simulink model "MSAP_avec_obs"  (R2021a)
settings: Solver=VariableStepAuto  StartTime=0.0  StopTime=10  FixedStep=0.00000001  RelTol=1e-4
values from neighbouring files (symbols this model uses):
  B = [ 1/Ld 0 ... (first row only)    [script_projet.m]
  C = [1 0 0 0 ... (first row only)    [script_projet.m]
  Cr = 5    [script_projet.m]
  f = 14*10^-5    (= 0.00014)    [script_projet.m]
  J = 11*10^-5    (= 0.00011)    [script_projet.m]
  Kid = 3*Rs/trd    (= 0.0014)    [script_projet.m]
  KiO = 3*f/tr2    (= 0.00011)    [script_projet.m]
  Kiq = 3*Rs/trq    (= 0.0028)    [script_projet.m]
  Kpd = 3*Ld/trd    (= 3.26666666667e-06)    [script_projet.m]
  KpO = 3*J/tr2*10^8    (= 8642.85714286)    [script_projet.m]
  Kpq = 3*Lq/trq    (= 1.30666666667e-05)    [script_projet.m]
  Ld = 0.0014    [script_projet.m]
  Lq = 0.0028    [script_projet.m]
  P = 4    [script_projet.m]
  phi_f = 0.12    [script_projet.m]
  Q = [1 0 0 0 ... (first row only)    [script_projet.m]
  R = [1 0 ... (first row only)    [script_projet.m]
  Rs = 0.6    [script_projet.m]
libraries: simulink x1
settings Model: Creator=atestard2020  LastModifiedBy=atestard2020
settings SolverCC: MaxConsecutiveMinStep=1000

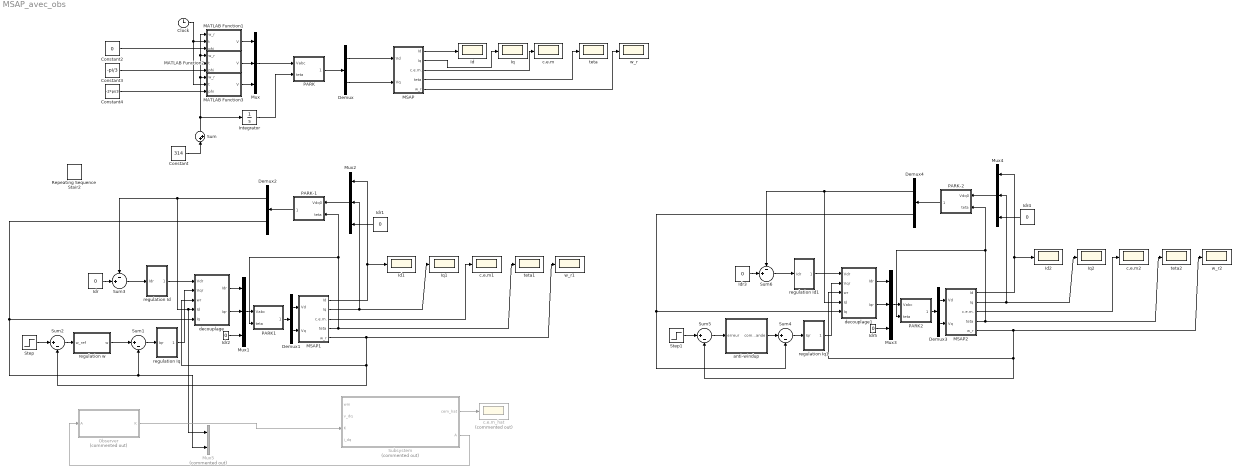
== system MSAP_avec_obs ==
  Clock : Clock
      settings: Decimation=1000000
  Constant : Constant  Value=314
  Constant2 : Constant  Value=0
  Constant3 : Constant  Value=-pi/3
  Constant4 : Constant  Value=-2*pi/3
  Demux{,1..4} (5 alike) : Demux  Outputs=2
  Id : Scope
  Id1 : Scope
  Id2 : Scope
  Idr{,1..5} (6 alike) : Constant  Value=0
  Integrator : Integrator
  Iq : Scope
  Iq1 : Scope
  Iq2 : Scope
  MATLAB Function1 : MATLAB Function  TreatAsAtomicUnit=on
  MATLAB Function2 : MATLAB Function  TreatAsAtomicUnit=on
  MATLAB Function3 : MATLAB Function  TreatAsAtomicUnit=on
  MSAP : Subsystem
  MSAP1 : Subsystem
  MSAP2 : Subsystem
  Mux{,1..4} (5 alike) : Mux  Inputs=3
  Mux5 : Mux  Commented=on  Inputs=2
  Observer : Subsystem  Commented=on
  PARK : MATLAB Function  TreatAsAtomicUnit=on
  PARK-1 : MATLAB Function  TreatAsAtomicUnit=on
  PARK-2 : MATLAB Function  TreatAsAtomicUnit=on
  PARK1 : MATLAB Function  TreatAsAtomicUnit=on
  PARK2 : MATLAB Function  TreatAsAtomicUnit=on
  Repeating Sequence Stair2 : simulink/Sources/Repeating Sequence Stair  OutValues=[3 1 4 2 1].'  tsamp=0.4  OutMin=[]  OutMax=[]  OutDataTypeStr=double  OutputDataTypeScalingMode=double  OutDataType=fixdt(0,8)  ConRadixGroup=Best Precision: Vector-wise  OutScaling=2^-12
  Step : Step  After=4  SampleTime=0
  Step1 : Step  SampleTime=0
  Subsystem : Subsystem  Commented=on
  Sum : Sum  Inputs=|++
  Sum{1..2,4..5} (4 alike) : Sum  Inputs=|+-
  Sum3 : Sum  Inputs=-+|
  Sum6 : Sum  Inputs=-+|
  anti-windup : Subsystem
  c.e.m : Scope
  c.e.m1 : Scope
  c.e.m2 : Scope
  c.e.m_hat : Scope  Commented=on
  decouplage : Subsystem
  decouplage1 : Subsystem
  regulation Id : Subsystem
  regulation Id1 : Subsystem
  regulation Iq : Subsystem
  regulation Iq1 : Subsystem
  regulation w : Subsystem
  teta : Scope
  teta1 : Scope
  teta2 : Scope
  w_r : Scope
  w_r1 : Scope
  w_r2 : Scope
  wires:
  MATLAB Function1/1(V) -> Mux/1
  MATLAB Function2/1(V) -> Mux/2
  Integrator/1 -> PARK/2(teta)
  Mux/1 -> PARK/1(Vabc)
  Demux/1 -> MSAP/1(Vd)
  MATLAB Function3/1(V) -> Mux/3
  PARK/1(TVdq0) -> Demux/1
  Demux/2 -> MSAP/2(Vq)
  MSAP/4(teta) -> teta/1
  MSAP/5(w_r) -> w_r/1
  MSAP/3(c.e.m.) -> c.e.m/1
  MSAP/2(Iq) -> Iq/1
  MSAP/1(Id) -> Id/1
  Constant2/1 -> MATLAB Function1/3(phi)
  Constant3/1 -> MATLAB Function2/3(phi)
  Constant4/1 -> MATLAB Function3/3(phi)
  Sum/1 -> Integrator/1, MATLAB Function1/1(w_r), MATLAB Function2/1(w_r), MATLAB Function3/1(w_r)
  Clock/1 -> MATLAB Function3/2(t), MATLAB Function2/2(t), MATLAB Function1/2(t)
  Constant/1 -> Sum/1
  Sum1/1 -> regulation Iq/1(Iqr)
  Sum3/1 -> regulation Id/1(Idr)
  Idr/1 -> Sum3/2
  Step/1 -> Sum2/1
  regulation Id/1(Vd1) -> decouplage/1(Vdr)
  regulation Iq/1(Vq1) -> decouplage/2(Vqr)
  Sum2/1 -> regulation w/1(w_ref)
  MSAP1/1(Id) -> Id1/1, Mux2/1
  MSAP1/2(Iq) -> Iq1/1, Mux2/2
  MSAP1/3(c.e.m.) -> c.e.m1/1
  MSAP1/5(w_r) -> w_r1/1, Sum2/2, decouplage/3(wr)
  regulation w/1(w) -> Sum1/1
  Mux1/1 -> PARK1/1(Vabc)
  PARK1/1(TVdq0) -> Demux1/1
  Demux1/1 -> MSAP1/1(Vd)
  Demux1/2 -> MSAP1/2(Vq)
  decouplage/1(Idr) -> Mux1/1
  decouplage/2(Iqr) -> Mux1/2
  PARK-1/1(TVabc) -> Demux2/1
  Mux2/1 -> PARK-1/1(Vdq0)
  Demux2/2 -> Mux5/2, Sum1/2, decouplage/5(Iq)
  Demux2/1 -> Mux5/1, decouplage/4(Id), Sum3/1
  Idr1/1 -> Mux2/3
  Idr2/1 -> Mux1/3
  MSAP1/4(teta) -> PARK1/2(teta), PARK-1/2(teta), teta1/1
  MSAP2/5(w_r) -> w_r2/1, Sum5/2, decouplage1/3(wr)
  MSAP2/2(Iq) -> Iq2/1, Mux4/2
  Idr4/1 -> Mux4/3
  decouplage1/1(Idr) -> Mux3/1
  Demux4/1 -> decouplage1/4(Id), Sum6/1
  decouplage1/2(Iqr) -> Mux3/2
  Mux3/1 -> PARK2/1(Vabc)
  MSAP2/4(teta) -> PARK2/2(teta), PARK-2/2(teta), teta2/1
  Mux4/1 -> PARK-2/1(Vdq0)
  Sum6/1 -> regulation Id1/1(Idr)
  Demux4/2 -> Sum4/2, decouplage1/5(Iq)
  PARK-2/1(TVabc) -> Demux4/1
  Demux3/2 -> MSAP2/2(Vq)
  Demux3/1 -> MSAP2/1(Vd)
  regulation Id1/1(Vd1) -> decouplage1/1(Vdr)
  MSAP2/1(Id) -> Id2/1, Mux4/1
  Sum4/1 -> regulation Iq1/1(Iqr)
  Sum5/1 -> anti-windup/1(erreur)
  Step1/1 -> Sum5/1
  Idr5/1 -> Mux3/3
  regulation Iq1/1(Vq1) -> decouplage1/2(Vqr)
  MSAP2/3(c.e.m.) -> c.e.m2/1
  Idr3/1 -> Sum6/2
  PARK2/1(TVdq0) -> Demux3/1
  anti-windup/1(commande) -> Sum4/1
  Subsystem/2(A) -> Observer/1(A)
  Observer/1(K) -> Subsystem/3(K)
  Subsystem/1(cem_hat) -> c.e.m_hat/1

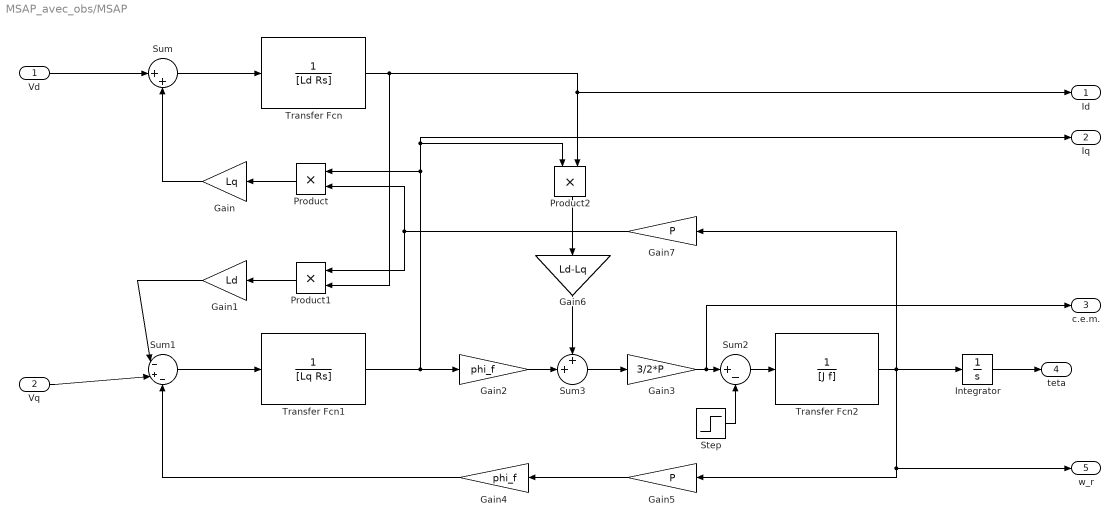
== system MSAP_avec_obs/MSAP ==
  Vd : Inport
  Vq : Inport  Port=2
  Gain : Gain  Gain=Lq
  Gain1 : Gain  Gain=Ld
  Gain2 : Gain  Gain=phi_f
  Gain3 : Gain  Gain=3/2*P
  Gain4 : Gain  Gain=phi_f
  Gain5 : Gain  Gain=P
  Gain6 : Gain  Gain=Ld-Lq
  Gain7 : Gain  Gain=P
  Integrator : Integrator
  Product : Product
  Product1 : Product
  Product2 : Product
  Step : Step  After=Cr  SampleTime=0
  Sum : Sum  Inputs=|++
  Sum1 : Sum  Inputs=|-+-
  Sum2 : Sum  Inputs=|+-
  Sum3 : Sum  Inputs=++|
  Transfer Fcn : TransferFcn  Denominator=[Ld Rs]
  Transfer Fcn1 : TransferFcn  Denominator=[Lq Rs]
  Transfer Fcn2 : TransferFcn  Denominator=[J f]
  Id : Outport
  Iq : Outport  Port=2
  c.e.m. : Outport  Port=3
  teta : Outport  Port=4
  w_r : Outport  Port=5
  wires:
  Transfer Fcn/1 -> Id/1, Product2/2, Product1/2
  Transfer Fcn1/1 -> Iq/1, Product2/1, Product/1, Gain2/1
  Gain3/1 -> c.e.m./1, Sum2/1
  Sum/1 -> Transfer Fcn/1
  Transfer Fcn2/1 -> Integrator/1, Gain7/1, w_r/1, Gain5/1
  Gain5/1 -> Gain4/1
  Gain2/1 -> Sum3/2
  Product2/1 -> Gain6/1
  Gain7/1 -> Product1/1, Product/2
  Gain6/1 -> Sum3/1
  Product1/1 -> Gain1/1
  Integrator/1 -> teta/1
  Product/1 -> Gain/1
  Vq/1 -> Sum1/2
  Sum1/1 -> Transfer Fcn1/1
  Gain1/1 -> Sum1/1
  Sum2/1 -> Transfer Fcn2/1
  Step/1 -> Sum2/2
  Gain4/1 -> Sum1/3
  Sum3/1 -> Gain3/1
  Gain/1 -> Sum/2
  Vd/1 -> Sum/1

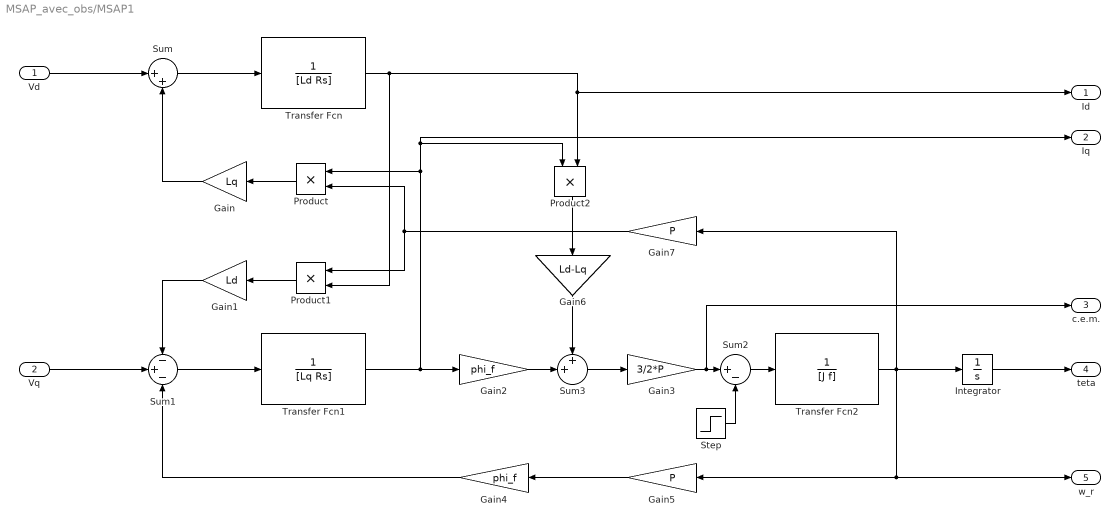
== system MSAP_avec_obs/MSAP1 ==
  Vd : Inport
  Vq : Inport  Port=2
  Gain : Gain  Gain=Lq
  Gain1 : Gain  Gain=Ld
  Gain2 : Gain  Gain=phi_f
  Gain3 : Gain  Gain=3/2*P
  Gain4 : Gain  Gain=phi_f
  Gain5 : Gain  Gain=P
  Gain6 : Gain  Gain=Ld-Lq
  Gain7 : Gain  Gain=P
  Integrator : Integrator
  Product : Product
  Product1 : Product
  Product2 : Product
  Step : Step  After=Cr  SampleTime=0
  Sum : Sum  Inputs=|++
  Sum1 : Sum  Inputs=-+-
  Sum2 : Sum  Inputs=|+-
  Sum3 : Sum  Inputs=++|
  Transfer Fcn : TransferFcn  Denominator=[Ld Rs]
  Transfer Fcn1 : TransferFcn  Denominator=[Lq Rs]
  Transfer Fcn2 : TransferFcn  Denominator=[J f]
  Id : Outport
  Iq : Outport  Port=2
  c.e.m. : Outport  Port=3
  teta : Outport  Port=4
  w_r : Outport  Port=5
  wires:
  Transfer Fcn/1 -> Id/1, Product2/2, Product1/2
  Transfer Fcn1/1 -> Iq/1, Product2/1, Product/1, Gain2/1
  Gain3/1 -> c.e.m./1, Sum2/1
  Sum/1 -> Transfer Fcn/1
  Transfer Fcn2/1 -> Integrator/1, Gain7/1, w_r/1, Gain5/1
  Gain5/1 -> Gain4/1
  Gain2/1 -> Sum3/2
  Product2/1 -> Gain6/1
  Gain7/1 -> Product1/1, Product/2
  Gain6/1 -> Sum3/1
  Product1/1 -> Gain1/1
  Integrator/1 -> teta/1
  Product/1 -> Gain/1
  Vq/1 -> Sum1/2
  Sum1/1 -> Transfer Fcn1/1
  Gain1/1 -> Sum1/1
  Sum2/1 -> Transfer Fcn2/1
  Step/1 -> Sum2/2
  Gain4/1 -> Sum1/3
  Sum3/1 -> Gain3/1
  Gain/1 -> Sum/2
  Vd/1 -> Sum/1

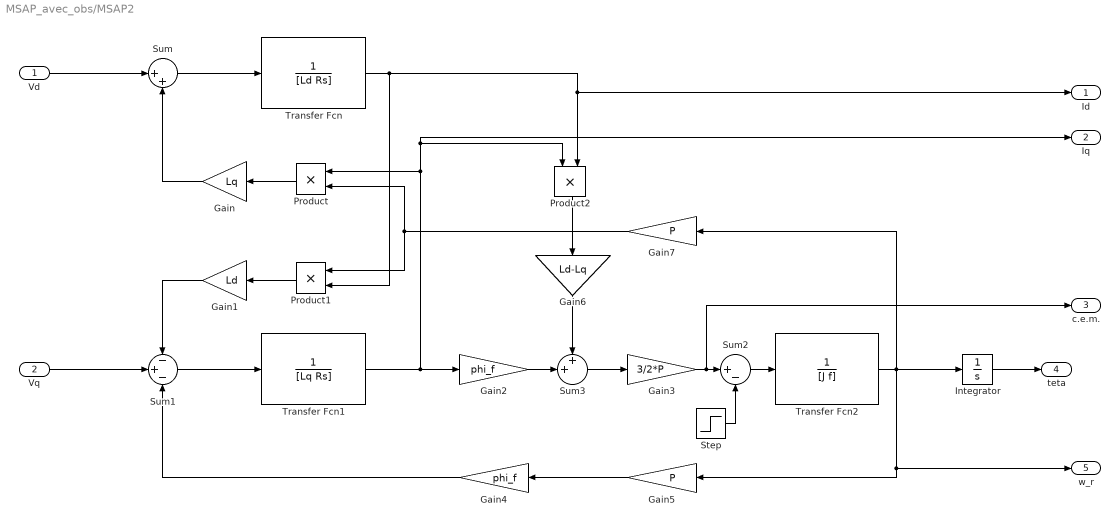
== system MSAP_avec_obs/MSAP2 ==
  Vd : Inport
  Vq : Inport  Port=2
  Gain : Gain  Gain=Lq
  Gain1 : Gain  Gain=Ld
  Gain2 : Gain  Gain=phi_f
  Gain3 : Gain  Gain=3/2*P
  Gain4 : Gain  Gain=phi_f
  Gain5 : Gain  Gain=P
  Gain6 : Gain  Gain=Ld-Lq
  Gain7 : Gain  Gain=P
  Integrator : Integrator
  Product : Product
  Product1 : Product
  Product2 : Product
  Step : Step  After=0  SampleTime=0
  Sum : Sum  Inputs=|++
  Sum1 : Sum  Inputs=-+-
  Sum2 : Sum  Inputs=|+-
  Sum3 : Sum  Inputs=++|
  Transfer Fcn : TransferFcn  Denominator=[Ld Rs]
  Transfer Fcn1 : TransferFcn  Denominator=[Lq Rs]
  Transfer Fcn2 : TransferFcn  Denominator=[J f]
  Id : Outport
  Iq : Outport  Port=2
  c.e.m. : Outport  Port=3
  teta : Outport  Port=4
  w_r : Outport  Port=5
  wires:
  Transfer Fcn/1 -> Id/1, Product2/2, Product1/2
  Transfer Fcn1/1 -> Iq/1, Product2/1, Product/1, Gain2/1
  Gain3/1 -> c.e.m./1, Sum2/1
  Sum/1 -> Transfer Fcn/1
  Transfer Fcn2/1 -> Integrator/1, Gain7/1, w_r/1, Gain5/1
  Gain5/1 -> Gain4/1
  Gain2/1 -> Sum3/2
  Product2/1 -> Gain6/1
  Gain7/1 -> Product1/1, Product/2
  Gain6/1 -> Sum3/1
  Product1/1 -> Gain1/1
  Integrator/1 -> teta/1
  Product/1 -> Gain/1
  Vq/1 -> Sum1/2
  Sum1/1 -> Transfer Fcn1/1
  Gain1/1 -> Sum1/1
  Sum2/1 -> Transfer Fcn2/1
  Step/1 -> Sum2/2
  Gain4/1 -> Sum1/3
  Sum3/1 -> Gain3/1
  Gain/1 -> Sum/2
  Vd/1 -> Sum/1

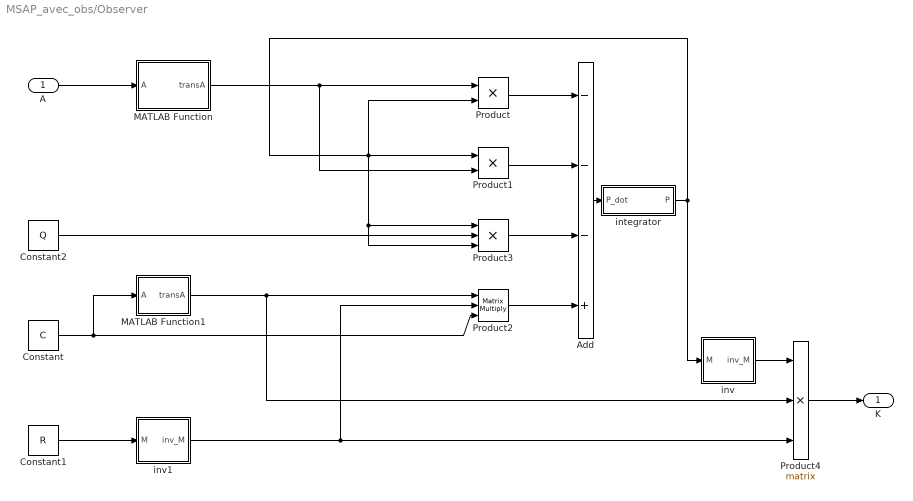
== system MSAP_avec_obs/Observer ==
  A : Inport  PortDimensions=[4;4]
  Add : Sum  Inputs=---+
  Constant : Constant  Value=C
  Constant1 : Constant  Value=R
  Constant2 : Constant  Value=Q
  MATLAB Function : MATLAB Function  TreatAsAtomicUnit=on
  MATLAB Function1 : MATLAB Function  TreatAsAtomicUnit=on
  Product : Product
  Product1 : Product
  Product2 : Product  Inputs=3  Multiplication=Matrix(*)
  Product3 : Product  Inputs=3
  Product4 : Product  Inputs=3  Multiplication=Matrix(*)
  integrator : Subsystem
  inv : MATLAB Function  TreatAsAtomicUnit=on
  inv1 : MATLAB Function  TreatAsAtomicUnit=on
  K : Outport
  wires:
  Product/1 -> Add/1
  Product1/1 -> Add/2
  Product3/1 -> Add/3
  Product2/1 -> Add/4
  MATLAB Function/1(transA) -> Product1/2, Product/1
  Add/1 -> integrator/1(P_dot)
  integrator/1(P) -> inv/1(M), Product1/1, Product/2, Product3/3, Product3/1
  Constant/1 -> Product2/3, MATLAB Function1/1(A)
  MATLAB Function1/1(transA) -> Product4/2, Product2/1
  inv/1(inv_M) -> Product4/1
  Constant1/1 -> inv1/1(M)
  inv1/1(inv_M) -> Product2/2, Product4/3
  Constant2/1 -> Product3/2
  Product4/1 -> K/1
  A/1 -> MATLAB Function/1(A)

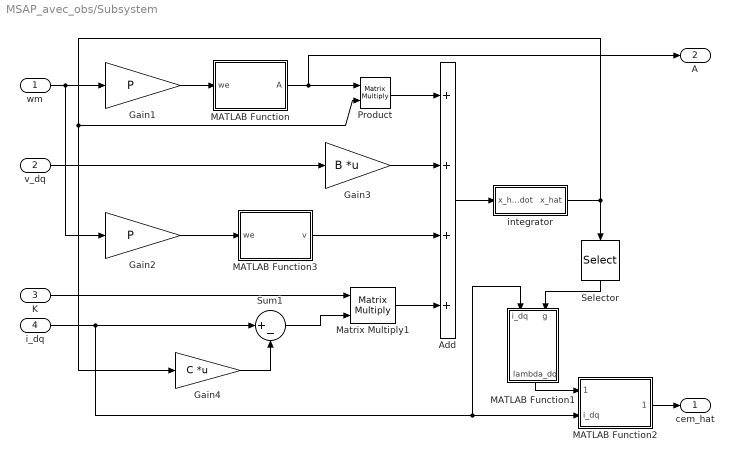
== system MSAP_avec_obs/Subsystem ==
  wm : Inport  PortDimensions=1
  v_dq : Inport  Port=2  PortDimensions=2
  K : Inport  Port=3  PortDimensions=[4;2]
  i_dq : Inport  Port=4  PortDimensions=2
  Add : Sum  Inputs=++++
  Gain1 : Gain  Gain=P
  Gain2 : Gain  Gain=P
  Gain3 : Gain  Gain=B  Multiplication=Matrix(K*u) (u vector)
  Gain4 : Gain  Gain=C  Multiplication=Matrix(K*u) (u vector)
  MATLAB Function : MATLAB Function  TreatAsAtomicUnit=on
  MATLAB Function1 : MATLAB Function  TreatAsAtomicUnit=on
  MATLAB Function2 : MATLAB Function  TreatAsAtomicUnit=on
  MATLAB Function3 : MATLAB Function  TreatAsAtomicUnit=on
  Matrix Multiply1 : Product  Multiplication=Matrix(*)
  Product : Product  Multiplication=Matrix(*)
  Selector : Selector  InputPortWidth=4  IndexOptions=Index vector (dialog)  Indices=[3 4]  OutputSizes=1
  Sum1 : Sum  Inputs=|+-
  integrator : Subsystem
  cem_hat : Outport
  A : Outport  Port=2
  wires:
  wm/1 -> Gain1/1, Gain2/1
  Gain1/1 -> MATLAB Function/1(we)
  MATLAB Function/1(A) -> A/1, Product/1
  Product/1 -> Add/1
  Gain3/1 -> Add/2
  Matrix Multiply1/1 -> Add/4
  Add/1 -> integrator/1(x_hat_dot)
  K/1 -> Matrix Multiply1/1
  Sum1/1 -> Matrix Multiply1/2
  i_dq/1 -> MATLAB Function1/1(i_dq), MATLAB Function2/2(i_dq), Sum1/1
  Gain4/1 -> Sum1/2
  MATLAB Function2/1(cem_hat) -> cem_hat/1
  MATLAB Function1/1(lambda_dq) -> MATLAB Function2/1(lambda_dq)
  Selector/1 -> MATLAB Function1/2(g)
  v_dq/1 -> Gain3/1
  MATLAB Function3/1(v) -> Add/3
  Gain2/1 -> MATLAB Function3/1(we)
  integrator/1(x_hat) -> Selector/1, Gain4/1, Product/2

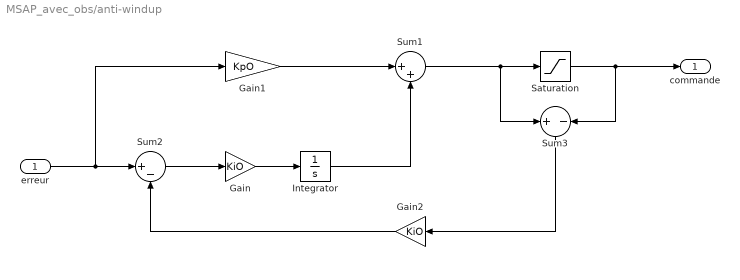
== system MSAP_avec_obs/anti-windup ==
  erreur : Inport
  Gain : Gain  Gain=KiO
  Gain1 : Gain  Gain=KpO
  Gain2 : Gain  Gain=KiO
  Integrator : Integrator
  Saturation : Saturate
  Sum1 : Sum  Inputs=|++
  Sum2 : Sum  Inputs=|+-
  Sum3 : Sum  Inputs=+|-
  commande : Outport
  wires:
  Sum1/1 -> Sum3/1, Saturation/1
  Saturation/1 -> Sum3/2, commande/1
  Integrator/1 -> Sum1/2
  Sum2/1 -> Gain/1
  Gain/1 -> Integrator/1
  Gain1/1 -> Sum1/1
  erreur/1 -> Gain1/1, Sum2/1
  Gain2/1 -> Sum2/2
  Sum3/1 -> Gain2/1

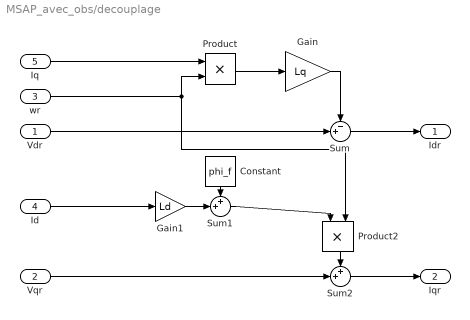
== system MSAP_avec_obs/decouplage ==
  Vdr : Inport
  Vqr : Inport  Port=2
  wr : Inport  Port=3
  Id : Inport  Port=4
  Iq : Inport  Port=5
  Constant : Constant  Value=phi_f
  Gain : Gain  Gain=Lq
  Gain1 : Gain  Gain=Ld
  Product : Product
  Product2 : Product
  Sum : Sum  Inputs=-+|
  Sum1 : Sum  Inputs=++|
  Sum2 : Sum  Inputs=++|
  Idr : Outport
  Iqr : Outport  Port=2
  wires:
  Vqr/1 -> Sum2/2
  Sum/1 -> Idr/1
  Sum2/1 -> Iqr/1
  Product/1 -> Gain/1
  wr/1 -> Product/2, Product2/2
  Iq/1 -> Product/1
  Gain/1 -> Sum/1
  Vdr/1 -> Sum/2
  Id/1 -> Gain1/1
  Gain1/1 -> Sum1/2
  Constant/1 -> Sum1/1
  Product2/1 -> Sum2/1
  Sum1/1 -> Product2/1

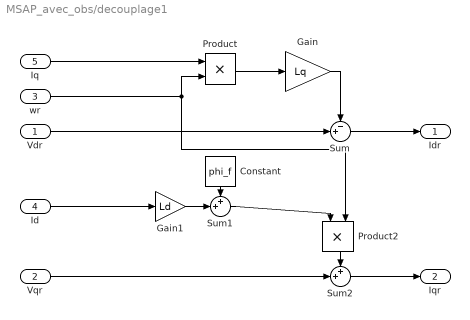
== system MSAP_avec_obs/decouplage1 ==
  Vdr : Inport
  Vqr : Inport  Port=2
  wr : Inport  Port=3
  Id : Inport  Port=4
  Iq : Inport  Port=5
  Constant : Constant  Value=phi_f
  Gain : Gain  Gain=Lq
  Gain1 : Gain  Gain=Ld
  Product : Product
  Product2 : Product
  Sum : Sum  Inputs=-+|
  Sum1 : Sum  Inputs=++|
  Sum2 : Sum  Inputs=++|
  Idr : Outport
  Iqr : Outport  Port=2
  wires:
  Vqr/1 -> Sum2/2
  Sum/1 -> Idr/1
  Sum2/1 -> Iqr/1
  Product/1 -> Gain/1
  wr/1 -> Product/2, Product2/2
  Iq/1 -> Product/1
  Gain/1 -> Sum/1
  Vdr/1 -> Sum/2
  Id/1 -> Gain1/1
  Gain1/1 -> Sum1/2
  Constant/1 -> Sum1/1
  Product2/1 -> Sum2/1
  Sum1/1 -> Product2/1

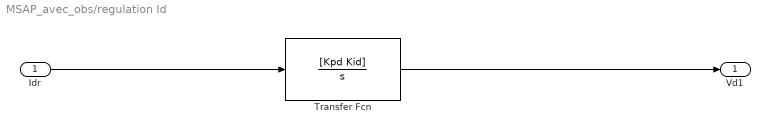
== system MSAP_avec_obs/regulation Id ==
  Idr : Inport
  Transfer Fcn : TransferFcn  Numerator=[Kpd Kid]  Denominator=[1 0]
  Vd1 : Outport
  wires:
  Idr/1 -> Transfer Fcn/1
  Transfer Fcn/1 -> Vd1/1

== system MSAP_avec_obs/regulation Id1 ==
  Idr : Inport
  Transfer Fcn : TransferFcn  Numerator=[Kpd Kid]  Denominator=[1 0]
  Vd1 : Outport
  wires:
  Idr/1 -> Transfer Fcn/1
  Transfer Fcn/1 -> Vd1/1

== system MSAP_avec_obs/regulation Iq ==
  Iqr : Inport
  Transfer Fcn : TransferFcn  Numerator=[Kpq Kiq]  Denominator=[1 0]
  Vq1 : Outport
  wires:
  Transfer Fcn/1 -> Vq1/1
  Iqr/1 -> Transfer Fcn/1

== system MSAP_avec_obs/regulation Iq1 ==
  Iqr : Inport
  Transfer Fcn : TransferFcn  Numerator=[Kpq Kiq]  Denominator=[1 0]
  Vq1 : Outport
  wires:
  Transfer Fcn/1 -> Vq1/1
  Iqr/1 -> Transfer Fcn/1

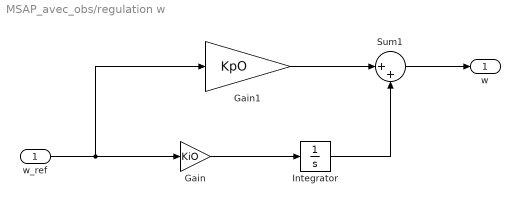
== system MSAP_avec_obs/regulation w ==
  w_ref : Inport
  Gain : Gain  Gain=KiO
  Gain1 : Gain  Gain=KpO
  Integrator : Integrator
  Sum1 : Sum  Inputs=|++
  w : Outport
  wires:
  Sum1/1 -> w/1
  Integrator/1 -> Sum1/2
  w_ref/1 -> Gain/1, Gain1/1
  Gain/1 -> Integrator/1
  Gain1/1 -> Sum1/1

== system MSAP_avec_obs/Observer/integrator ==
  P_dot : Inport
  Integrator1 : Integrator
  P : Outport
  wires:
  P_dot/1 -> Integrator1/1
  Integrator1/1 -> P/1

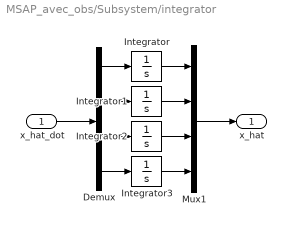
== system MSAP_avec_obs/Subsystem/integrator ==
  x_hat_dot : Inport
  Demux : Demux
  Integrator{,1..3} (4 alike) : Integrator
  Mux1 : Mux
  x_hat : Outport
  wires:
  x_hat_dot/1 -> Demux/1
  Mux1/1 -> x_hat/1
  Integrator1/1 -> Mux1/2
  Demux/2 -> Integrator1/1
  Demux/3 -> Integrator2/1
  Integrator2/1 -> Mux1/3
  Demux/4 -> Integrator3/1
  Integrator3/1 -> Mux1/4
  Demux/1 -> Integrator/1
  Integrator/1 -> Mux1/1

== matlab function MSAP_avec_obs/Subsystem/MATLAB Function2 ==
  data: lambda_dq input; cem_hat output; i_dq input
function cem_hat = fcn(lambda_dq, i_dq)
P=4;
cem_hat = (3/2)*P*(lambda_dq(1)*i_dq(2)-lambda_dq(2)*i_dq(1));

== matlab function MSAP_avec_obs/Subsystem/MATLAB Function3 ==
  data: we input; v output
function v = fcn(we)
Lq = 0.0028 ; %Inductance linéaire du stator selon l'axe q (H)
phi_f = 0.12 ; %flux d'aimant permanent (Wb)
v = [ 0;
    -we*phi_f/Lq
    0;
    0;];

== matlab function MSAP_avec_obs/Observer/MATLAB Function ==
  data: A input; transA output
function transA = fcn(A)

transA = A';

== matlab function MSAP_avec_obs/Observer/MATLAB Function1 ==
  data: A input; transA output
function transA = fcn(A)

transA = A';

== matlab function MSAP_avec_obs/PARK ==
  data: Vabc input; TVdq0 output; teta input
function TVdq0 = T(Vabc,teta)
T=2/3*[ cos(teta) cos(teta-2*pi/3) cos(teta+2*pi/3) ;
        sin(teta) sin(teta-2*pi/3) sin(teta+2*pi/3) ;
        1/2         1/2                 1/2         ;];
TVdq0bis = T*Vabc;
TVdq0 = [TVdq0bis(1) ; TVdq0bis(2)];

== matlab function MSAP_avec_obs/MATLAB Function2 ==
  data: w_r input; t input; V output; phi input
function V = fcn(w_r,t,phi)
V=220*sin(w_r*t+phi);

== matlab function MSAP_avec_obs/MATLAB Function3 ==
  data: w_r input; t input; V output; phi input
function V = fcn(w_r,t,phi)
V=220*sin(w_r*t+phi);

== matlab function MSAP_avec_obs/PARK-1 ==
  data: Vdq0 input; TVabc output; teta input
function TVabc = Tinv(Vdq0,teta)
T=[ cos(teta)        sin(teta)        1 ;
    cos(teta-2*pi/3) sin(teta-2*pi/3) 1 ;
    cos(teta+2*pi/3) sin(teta+2*pi/3) 1 ;];
TVabcbis = T*Vdq0;
TVabc = [TVabcbis(1) ; TVabcbis(2)];

== matlab function MSAP_avec_obs/PARK1 ==
  data: Vabc input; TVdq0 output; teta input
function TVdq0 = T(Vabc,teta)
T=2/3*[ cos(teta) cos(teta-2*pi/3) cos(teta+2*pi/3) ;
        sin(teta) sin(teta-2*pi/3) sin(teta+2*pi/3) ;
        1/2         1/2                 1/2         ;];
TVdq0bis = T*Vabc;
TVdq0 = [TVdq0bis(1) ; TVdq0bis(2)];

== matlab function MSAP_avec_obs/PARK-2 ==
  data: Vdq0 input; TVabc output; teta input
function TVabc = Tinv(Vdq0,teta)
T=[ cos(teta)        sin(teta)        1 ;
    cos(teta-2*pi/3) sin(teta-2*pi/3) 1 ;
    cos(teta+2*pi/3) sin(teta+2*pi/3) 1 ;];
TVabcbis = T*Vdq0;
TVabc = [TVabcbis(1) ; TVabcbis(2)];

== matlab function MSAP_avec_obs/PARK2 ==
  data: Vabc input; TVdq0 output; teta input
function TVdq0 = T(Vabc,teta)
T=2/3*[ cos(teta) cos(teta-2*pi/3) cos(teta+2*pi/3) ;
        sin(teta) sin(teta-2*pi/3) sin(teta+2*pi/3) ;
        1/2         1/2                 1/2         ;];
TVdq0bis = T*Vabc;
TVdq0 = [TVdq0bis(1) ; TVdq0bis(2)];

== matlab function MSAP_avec_obs/Observer/inv ==
  data: M input; inv_M output
function inv_M = inv(M)
inv_M = M^-1;

== matlab function MSAP_avec_obs/Observer/inv1 ==
  data: M input; inv_M output
function inv_M = inv(M)
inv_M = M^-1;

== matlab function MSAP_avec_obs/MATLAB Function1 ==
  data: w_r input; t input; V output; phi input
function V = fcn(w_r,t,phi)
V=220*sin(w_r*t+phi);

== matlab function MSAP_avec_obs/Subsystem/MATLAB Function ==
  data: we input; A output
function A = fcn(we)
Rs = 0.6 ; %Résistance du stator (Ohm)
Ld = 0.0014 ; %Inductance linéaire du stator selon l'axe d (H)
Lq = 0.0028 ; %Inductance linéaire du stator selon l'axe q (H)
A = [ -Rs/Ld we*Lq/Ld 0 -we*Lq/Ld ;
      -we*Ld/Lq -Rs/Lq we*Ld/Lq 0;
      0 0 0 0;
      0 0 0 0;];

== matlab function MSAP_avec_obs/Subsystem/MATLAB Function1 ==
  data: i_dq input; lambda_dq output; g input
function lambda_dq = fcn(i_dq, g)
phi_f = 0.12 ; %flux d'aimant permanent (Wb)
Ld = 0.0014 ; %Inductance linéaire du stator selon l'axe d (H)
Lq = 0.0028 ; %Inductance linéaire du stator selon l'axe q (H)
lambda_d = phi_f + Ld*(i_dq(1)-g(1));
lambda_q = Lq*(i_dq(1) - g(2));
lambda_dq = [lambda_d lambda_q];
